simulink model "bicycle_sim3"  (Simulink 8.7)
settings: Solver=VariableStepAuto  SolverMode=SingleTasking  StartTime=0.0  StopTime=489.5  RelTol=1e-3
values from neighbouring files (symbols this model uses):
  a = 4    [bicycle.m]
  d = 0.03    [bicycle.m]
  Kp = 7    [bicycle.m]
  theta0 = pi/2    (= 1.57079632679)    [bicycle.m]
  w = 0.1    [bicycle.m]
  x0 = a    (= 4)    [bicycle.m]
  y0 = 0    [bicycle.m]
undefined symbols (not defined in the file or in its folder): K_th, K_x, K_y
libraries: simulink_extras x2
settings Model: Creator=olivier  LastModifiedBy=sanjy
settings SolverCC: ZeroCrossAlgorithm=Adaptive
settings DataIOCC: LimitDataPoints=off  SaveFormat=Dataset
settings DebuggingCC: UnderspecifiedInitializationDetection=Simplified  MergeDetectMultiDrivingBlocksExec=error  MaskedZcDiagnostic=none  SFUnexpectedBacktrackingDiag=error  SFNoUnconditionalDefaultTransitionDiag=error
settings HardwareCC: ProdBitPerPointer=64  ProdLargestAtomicFloat=Float  ProdIntDivRoundTo=Zero  ProdEndianess=LittleEndian  ProdWordSize=64  ProdHWDeviceType=Intel->x86-64 (Windows64)
settings ModelReferenceCC: PropagateSignalLabelsOutOfModel=on
settings SFSimCC: SimUseLocalCustomCode=on
settings RTWCC: RTWUseLocalCustomCode=on
settings GRTTargetCC: TargetLangStandard=C99 (ISO)  GeneratePreprocessorConditionals=Use local settings
settings ConfigComp: CovMetricSettings=dwe  CovHtmlReporting=off  CovSaveCumulativeToWorkspaceVar=off  CovSaveSingleToWorkspaceVar=off  CovModelRefEnable=off  CovExternalEMLEnable=on

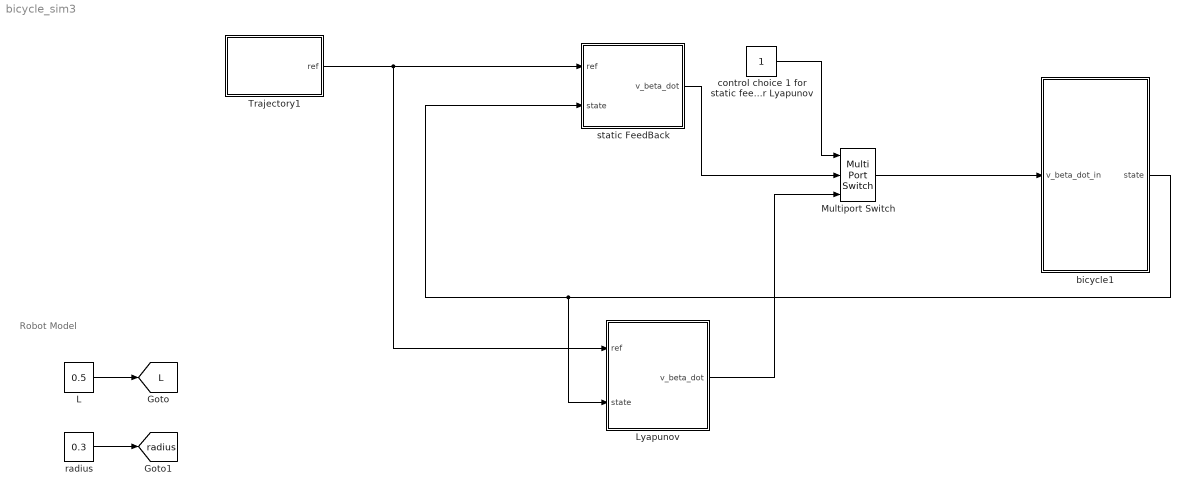
== system bicycle_sim3 ==
  note: Robot Model
  L : Constant  Value=0.5
  Lyapunov : Subsystem
  Multiport Switch : MultiPortSwitch  Inputs=2
  Trajectory1 : Subsystem  TreatAsAtomicUnit=on
  bicycle1 : Subsystem  mask{L_error=0, radius_error=0, omega_max=100, beta_max=6.5, beta_dot_max=50}
      mask prompts: L_error "L error in percent"; radius_error "Radius error in percent"; omega_max "Max Rotation Velocity"; beta_max "Max Orientation"; beta_dot_max "Max Orientation Velocity"
  control choice 1 for static feedback 2 for Lyapunov : Constant
  radius : Constant  Value=0.3
  static FeedBack : Subsystem
  tag scope: L=global, radius=global
  wires:
  static FeedBack/1(v_beta_dot) -> Multiport Switch/2
  L/1 -> [L]
  Trajectory1/1(ref) -> static FeedBack/1(ref), Lyapunov/1(ref)
  bicycle1/1(state) -> Lyapunov/2(state), static FeedBack/2(state)
  control choice 1 for static feedback 2 for Lyapunov/1 -> Multiport Switch/1
  Multiport Switch/1 -> bicycle1/1(v_beta_dot_in)
  Lyapunov/1(v_beta_dot) -> Multiport Switch/3
  radius/1 -> [radius]

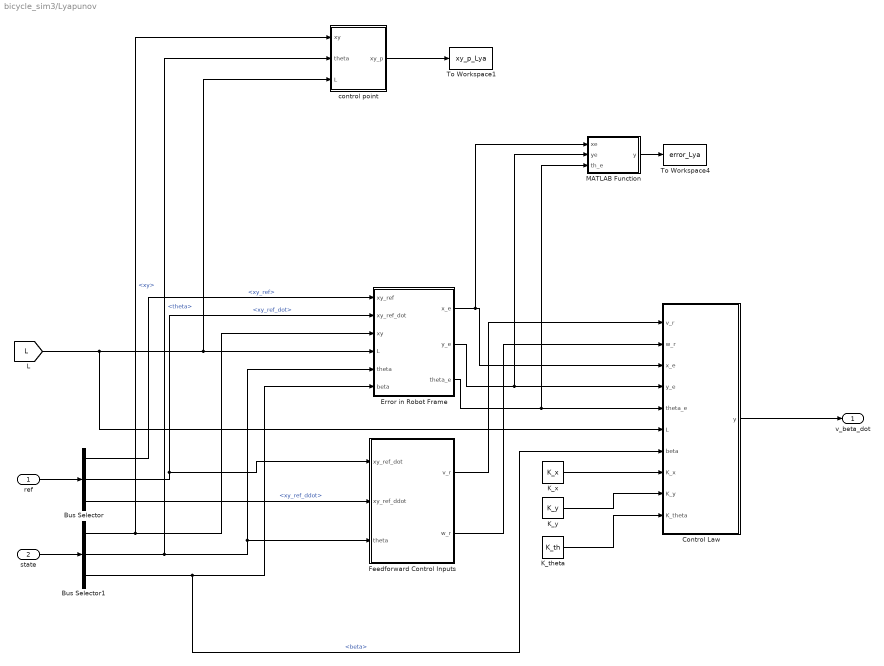
== system bicycle_sim3/Lyapunov ==
  ref : Inport
  state : Inport  Port=2
  Bus Selector : BusSelector  OutputSignals=xy_ref,xy_ref_dot,xy_ref_ddot
  Bus Selector1 : BusSelector  OutputSignals=xy,theta,beta
  Control Law : MATLAB Function  TreatAsAtomicUnit=on
  Error in Robot Frame : MATLAB Function  TreatAsAtomicUnit=on
  Feedforward Control Inputs : MATLAB Function  TreatAsAtomicUnit=on
  K_theta : Constant  Value=K_th
  K_x : Constant  Value=K_x
  K_y : Constant  Value=K_y
  MATLAB Function : MATLAB Function  TreatAsAtomicUnit=on
  To Workspace1 : ToWorkspace  VariableName=xy_p_Lya  SampleTime=-1
      settings: Save2DSignal=2-D array (concatenate along first dimension)
  To Workspace4 : ToWorkspace  VariableName=error_Lya  SampleTime=-1
      settings: Save2DSignal=2-D array (concatenate along first dimension)
  control point : MATLAB Function  TreatAsAtomicUnit=on
  v_beta_dot : Outport
  wires:
  ref/1 -> Bus Selector/1
  state/1 -> Bus Selector1/1
  Bus Selector/1 -> Error in Robot Frame/1(xy_ref)  "<xy_ref>"
  Bus Selector/2 -> Error in Robot Frame/2(xy_ref_dot), Feedforward Control Inputs/1(xy_ref_dot)  "<xy_ref_dot>"
  Bus Selector1/1 -> control point/1(xy), Error in Robot Frame/3(xy)  "<xy>"
  [L] -> Control Law/6(L), control point/3(L), Error in Robot Frame/4(L)
  Bus Selector1/2 -> control point/2(theta), Feedforward Control Inputs/3(theta), Error in Robot Frame/5(theta)  "<theta>"
  Bus Selector1/3 -> Control Law/7(beta), Error in Robot Frame/6(beta)  "<beta>"
  Bus Selector/3 -> Feedforward Control Inputs/2(xy_ref_ddot)  "<xy_ref_ddot>"
  Feedforward Control Inputs/1(v_r) -> Control Law/1(v_r)
  Feedforward Control Inputs/2(w_r) -> Control Law/2(w_r)
  Error in Robot Frame/1(x_e) -> MATLAB Function/1(xe), Control Law/3(x_e)
  Error in Robot Frame/2(y_e) -> MATLAB Function/2(ye), Control Law/4(y_e)
  Error in Robot Frame/3(theta_e) -> MATLAB Function/3(th_e), Control Law/5(theta_e)
  K_x/1 -> Control Law/8(K_x)
  K_y/1 -> Control Law/9(K_y)
  K_theta/1 -> Control Law/10(K_theta)
  Control Law/1(y) -> v_beta_dot/1
  MATLAB Function/1(y) -> To Workspace4/1
  control point/1(xy_p) -> To Workspace1/1

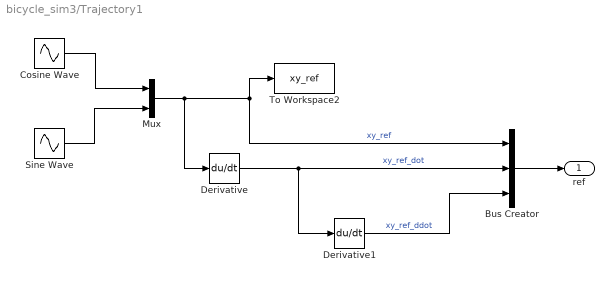
== system bicycle_sim3/Trajectory1 ==
  Bus Creator : BusCreator  Inputs=3
  Cosine Wave : Sin  Amplitude=a  Frequency=w  Phase=pi/2  SampleTime=0
  Derivative : Derivative
  Derivative1 : Derivative
  Mux : Mux  Inputs=2
  "Sine Wave " : Sin  Amplitude=a  Frequency=w  SampleTime=0
  To Workspace2 : ToWorkspace  VariableName=xy_ref  SampleTime=-1
      settings: Save2DSignal=2-D array (concatenate along first dimension)
  ref : Outport
  wires:
  Bus Creator/1 -> ref/1
  Mux/1 -> Derivative/1, Bus Creator/1, To Workspace2/1  "xy_ref"
  Derivative/1 -> Bus Creator/2, Derivative1/1  "xy_ref_dot"
  Derivative1/1 -> Bus Creator/3  "xy_ref_ddot"
  "Sine Wave "/1 -> Mux/2
  Cosine Wave/1 -> Mux/1

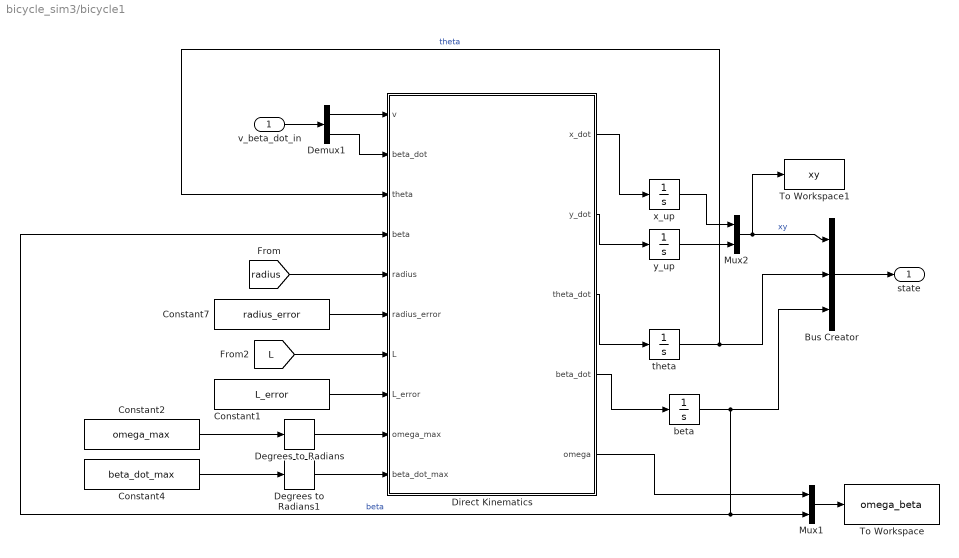
== system bicycle_sim3/bicycle1 ==
  v_beta_dot_in : Inport
  Bus Creator : BusCreator  Inputs=3
  Constant1 : Constant  Value=L_error
  Constant2 : Constant  Value=omega_max
  Constant4 : Constant  Value=beta_dot_max
  Constant7 : Constant  Value=radius_error
  Degrees to Radians : simulink_extras/Transformations/Degrees to Radians
  Degrees to Radians1 : simulink_extras/Transformations/Degrees to Radians
  Demux1 : Demux  Outputs=2
  Direct Kinematics : MATLAB Function  TreatAsAtomicUnit=on
  Mux1 : Mux  Inputs=2
  Mux2 : Mux  Inputs=2
  To Workspace : ToWorkspace  VariableName=omega_beta  SampleTime=-1
      settings: Save2DSignal=2-D array (concatenate along first dimension)
  To Workspace1 : ToWorkspace  VariableName=xy  SampleTime=-1
      settings: Save2DSignal=2-D array (concatenate along first dimension)
  beta : Integrator  LimitOutput=on  UpperSaturationLimit=beta_max*pi/180  LowerSaturationLimit=-beta_max*pi/180
  theta : Integrator  InitialCondition=theta0
  x_up : Integrator  InitialCondition=x0
  y_up : Integrator  InitialCondition=y0
  state : Outport
  wires:
  Direct Kinematics/2(y_dot) -> y_up/1
  Direct Kinematics/1(x_dot) -> x_up/1
  x_up/1 -> Mux2/1
  y_up/1 -> Mux2/2
  Mux2/1 -> Bus Creator/1, To Workspace1/1  "xy"
  Bus Creator/1 -> state/1
  v_beta_dot_in/1 -> Demux1/1
  Demux1/1 -> Direct Kinematics/1(v)
  [L] -> Direct Kinematics/7(L)
  Constant1/1 -> Direct Kinematics/8(L_error)
  Constant7/1 -> Direct Kinematics/6(radius_error)
  Direct Kinematics/3(theta_dot) -> theta/1
  Direct Kinematics/4(beta_dot) -> beta/1
  theta/1 -> Direct Kinematics/3(theta), Bus Creator/2  "theta"
  beta/1 -> Direct Kinematics/4(beta), Mux1/2, Bus Creator/3  "beta"
  Constant2/1 -> Degrees to Radians/1
  Constant4/1 -> Degrees to Radians1/1
  Direct Kinematics/5(omega) -> Mux1/1
  Mux1/1 -> To Workspace/1
  Demux1/2 -> Direct Kinematics/2("beta_dot ")
  Degrees to Radians/1 -> Direct Kinematics/9(omega_max)
  Degrees to Radians1/1 -> Direct Kinematics/10(beta_dot_max)
  [radius] -> Direct Kinematics/5(radius)

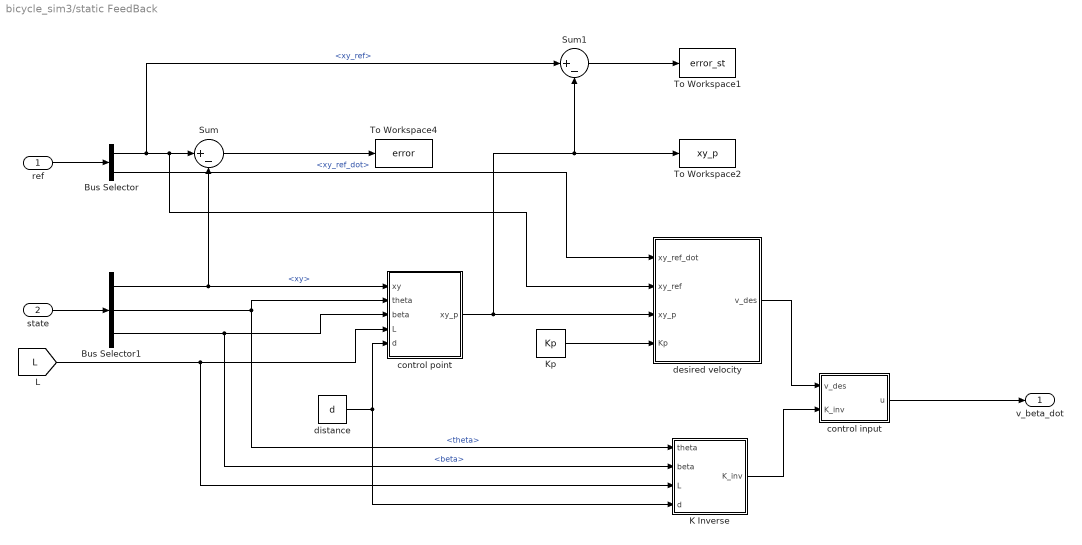
== system bicycle_sim3/static FeedBack ==
  ref : Inport
  state : Inport  Port=2
  Bus Selector : BusSelector  OutputSignals=xy_ref,xy_ref_dot
  Bus Selector1 : BusSelector  OutputSignals=xy,theta,beta
  K Inverse : MATLAB Function  TreatAsAtomicUnit=on
  Kp : Constant  Value=Kp
  Sum : Sum  Inputs=|+-
  Sum1 : Sum  Inputs=|+-
  To Workspace1 : ToWorkspace  VariableName=error_st  SampleTime=-1
      settings: Save2DSignal=2-D array (concatenate along first dimension)
  To Workspace2 : ToWorkspace  VariableName=xy_p  SampleTime=-1
      settings: Save2DSignal=2-D array (concatenate along first dimension)
  To Workspace4 : ToWorkspace  VariableName=error  SampleTime=-1
      settings: Save2DSignal=2-D array (concatenate along first dimension)
  control input : MATLAB Function  TreatAsAtomicUnit=on
  control point : MATLAB Function  TreatAsAtomicUnit=on
  desired velocity : MATLAB Function  TreatAsAtomicUnit=on
  distance : Constant  Value=d
  v_beta_dot : Outport
  wires:
  Sum/1 -> To Workspace4/1
  ref/1 -> Bus Selector/1
  state/1 -> Bus Selector1/1
  Bus Selector/1 -> Sum1/1, desired velocity/2(xy_ref), Sum/1  "<xy_ref>"
  Bus Selector1/1 -> Sum/2, control point/1(xy)  "<xy>"
  Bus Selector1/3 -> K Inverse/2(beta), control point/3(beta)  "<beta>"
  Bus Selector/2 -> desired velocity/1(xy_ref_dot)  "<xy_ref_dot>"
  Bus Selector1/2 -> control point/2(theta), K Inverse/1(theta)  "<theta>"
  [L] -> K Inverse/3(L), control point/4(L)
  distance/1 -> control point/5(d), K Inverse/4(d)
  control point/1(xy_p) -> Sum1/2, To Workspace2/1, desired velocity/3(xy_p)
  Kp/1 -> desired velocity/4(Kp)
  desired velocity/1(v_des) -> control input/1(v_des)
  K Inverse/1(K_inv) -> control input/2(K_inv)
  control input/1(u) -> v_beta_dot/1
  Sum1/1 -> To Workspace1/1

== matlab function static FeedBack/desired velocity ==
  data: xy_ref_dot input double; v_des output double; xy_ref input double; xy_p input double; Kp input double
function v_des = fcn(xy_ref_dot,xy_ref,xy_p,Kp)

v_des = xy_ref_dot + Kp*(xy_ref-xy_p);

== matlab function static FeedBack/control point ==
  data: xy input double; xy_p output double; theta input double; beta input double; L input double; d input double
function xy_p = fcn(xy,theta,beta,L,d)

x_p= xy(1) + L*cos(theta) + d*cos(theta+beta);
y_p= xy(end) + L*sin(theta) + d*sin(theta+beta);

xy_p=[x_p;y_p];

== matlab function static FeedBack/K Inverse ==
  data: theta input double; K_inv output double; beta input double; L input double; d input double
function K_inv = fcn(theta, beta, L, d)

%K = [L*cos(beta)*cos(theta)-(L*sin(theta)+d*sin(theta+beta))*sin(beta) -d*sin(theta+beta);
%     L*cos(beta)*sin(theta)+(L*cos(theta)+d*cos(theta+beta))*sin(beta) d*cos(theta+beta) ];

K = [ cos(theta+beta)-(d/L)*sin(beta)*sin(theta+beta) -d*sin(theta+beta);
      sin(theta+beta)+(d/L)*sin(beta)*cos(theta+beta) +d*cos(theta+beta)];

K_inv = inv(K);

== matlab function static FeedBack/control input ==
  data: v_des input double; u output double size=[2]; K_inv input double
function u = fcn(v_des,K_inv)

u = K_inv*v_des;

== matlab function Lyapunov/Error in Robot Frame ==
  data: xy_ref input double; x_e output double; xy_ref_dot input double; xy input double; L input double; theta input double; beta input double; y_e output double; theta_e output double
function [x_e,y_e,theta_e] = fcn(xy_ref,xy_ref_dot,xy,L,theta,beta)


x_e = cos(theta)*(xy_ref(1)-xy(1)-L*cos(theta)) + sin(theta)*(xy_ref(2)-xy(end)-L*sin(theta));
y_e = -sin(theta)*(xy_ref(1)-xy(1)-L*cos(theta)) + cos(theta)*(xy_ref(2)-xy(end)-L*sin(theta));

var = atan2(xy_ref_dot(2),xy_ref_dot(1)) - theta - beta;
theta_e = var - 2*pi*floor((var + pi)/(2*pi));

== matlab function Lyapunov/Feedforward Control Inputs ==
  data: xy_ref_dot input double; v_r output double; xy_ref_ddot input double; w_r output double; theta input double
function [v_r,w_r] = fcn(xy_ref_dot,xy_ref_ddot, theta)


v_r = xy_ref_dot(1)*cos(theta) + xy_ref_dot(2)*sin(theta);
if v_r==0
    w_r=0;
else
w_r = (xy_ref_dot(1)*xy_ref_ddot(2) - xy_ref_ddot(1)*xy_ref_dot(2))/(v_r^2);
end

== matlab function Lyapunov/Control Law ==
  data: v_r input double; y output double; w_r input double; x_e input double; y_e input double; theta_e input double; L input double; beta input double; K_x input double; K_y input double; K_theta input double
function y = fcn(v_r,w_r,x_e,y_e,theta_e,L,beta,K_x,K_y,K_theta)

if theta_e ==0
    w = w_r + K_y*y_e*v_r;
else
    w = w_r + K_y*y_e*v_r*(sin(theta_e)/(theta_e)) + K_theta*theta_e;
end

v = v_r*cos(theta_e) + K_x*x_e;


beta_dot = w - (v/L)*sin(beta);

y = [v,beta_dot];

== matlab function bicycle1/Direct Kinematics ==
  data: v input double; beta_dot input double; x_dot output double; theta input double; beta input double; radius input double; radius_error input double; L input double; L_error input double; omega_max input double; beta_dot_max input double; y_dot output double; theta_dot output double; beta_dot output double; omega output double
function [x_dot, y_dot, theta_dot, beta_dot, omega]  = dk(v, beta_dot, theta, beta, radius, radius_error, L, L_error, omega_max, beta_dot_max)

% commanded wheel rotation velocity
omega = v/radius;
omega = max(-omega_max, min(omega, omega_max));

% actual linear velocity
v = (1+radius_error*0.01)*radius * omega;

% actual L value
L = (1+L_error*0.01)*L;

x_dot = v*cos(theta)*cos(beta);
y_dot = v*sin(theta)*cos(beta);
theta_dot = v*sin(beta)/L;
beta_dot = max(-beta_dot_max, min(beta_dot, beta_dot_max));

== matlab function Lyapunov/MATLAB Function ==
  data: xe input double; y output double; ye input double; th_e input double
function y = fcn(xe,ye,th_e)

y = [ xe, ye,th_e];

== matlab function Lyapunov/control point ==
  data: xy input double; xy_p output double; theta input double; L input double
function xy_p = fcn(xy,theta,L)

x_p= xy(1) + L*cos(theta);
y_p= xy(end) + L*sin(theta);

xy_p=[x_p;y_p];
